simulink model "ProjektSim"  (R2018a)
settings: Solver=VariableStepAuto  StartTime=0.0  StopTime=50000  MaxStep=10  RelTol=1e-3
values from neighbouring files (symbols this model uses):
  Cp = 1000    [Projekt.m]
  Cvp = Cp * Rp * Vp    [Projekt.m]
  Cvw = Cp * Rp * Vw    [Projekt.m]
  Czas_skok = 5000    [Projekt.m]
  dFk = 0    [Projekt.m]
  dTg = -4    [Projekt.m]
  dTkz = 0    [Projekt.m]
  dTzew = -10    [Projekt.m]
  Fk0 = FkN    [Projekt.m]
  k1 = (Cp * Rp * FkN * (TkzN - TwewN) - kp * (TwewN - TpN)) / (TwewN - TzewN)    [Projekt.m]
  k2 = kp * (TwewN - TpN) / (TpN - TgN)    [Projekt.m]
  kp = Pr * Cp * Rp * FkN * (TkzN - TwewN) / (TwewN - TpN)    [Projekt.m]
  Rp = 1.2    [Projekt.m]
  Tg0 = TgN    (= -5)    [Projekt.m]
  Tkz0 = TkzN    (= 35)    [Projekt.m]
  Tp0 = (kp * Twew0 + k2 * Tg0) / (k2 + kp)    [Projekt.m]
  Twew0 = (Cp * Rp * Fk0 * Tkz0 + k1 * Tzew0 + k2 * kp * Tg0 / (k2 + kp)) / (Cp * Rp * Fk0 + k1 + kp - kp * kp / (k2 + kp))    [Projekt.m]
  Tzew0 = TzewN    (= -20)    [Projekt.m]
settings Model: Creator=aplov  LastModifiedBy=aplov

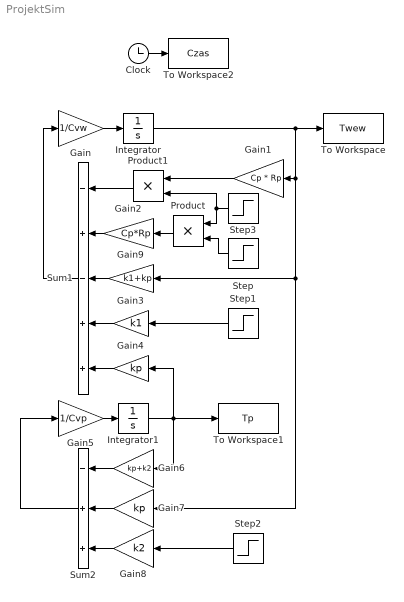
== system ProjektSim ==
  Clock : Clock
  Gain : Gain  Gain=1/Cvw
  Gain1 : Gain  Gain=Cp * Rp
  Gain2 : Gain  Gain=Cp*Rp
  Gain3 : Gain  Gain=k1
  Gain4 : Gain  Gain=kp
  Gain5 : Gain  Gain=1/Cvp
  Gain6 : Gain  Gain=kp+k2
  Gain7 : Gain  Gain=kp
  Gain8 : Gain  Gain=k2
  Gain9 : Gain  Gain=k1+kp
  Integrator : Integrator  InitialCondition=Twew0
  Integrator1 : Integrator  InitialCondition=Tp0
  Product : Product
  Product1 : Product
  Step : Step  Time=Czas_skok  Before=Tkz0  After=Tkz0 + dTkz  SampleTime=0
  Step1 : Step  Time=Czas_skok  Before=Tzew0  After=Tzew0 + dTzew  SampleTime=0
  Step2 : Step  Time=Czas_skok  Before=Tg0  After=Tg0 + dTg  SampleTime=0
  Step3 : Step  Time=Czas_skok  Before=Fk0  After=Fk0 + dFk  SampleTime=0
  Sum1 : Sum  Inputs=-+-++
  Sum2 : Sum  Inputs=-++
  To Workspace : ToWorkspace  VariableName=Twew  SampleTime=-1
  To Workspace1 : ToWorkspace  VariableName=Tp  SampleTime=-1
  To Workspace2 : ToWorkspace  VariableName=Czas  SampleTime=-1
  wires:
  Gain/1 -> Integrator/1
  Sum1/1 -> Gain/1
  Gain2/1 -> Sum1/2
  Gain3/1 -> Sum1/4
  Step1/1 -> Gain3/1
  Gain4/1 -> Sum1/5
  Integrator1/1 -> Gain6/1, To Workspace1/1, Gain4/1
  Gain5/1 -> Integrator1/1
  Sum2/1 -> Gain5/1
  Gain6/1 -> Sum2/1
  Gain7/1 -> Sum2/2
  Integrator/1 -> To Workspace/1, Gain7/1, Gain9/1, Gain1/1
  Gain8/1 -> Sum2/3
  Step2/1 -> Gain8/1
  Clock/1 -> To Workspace2/1
  Product/1 -> Gain2/1
  Step3/1 -> Product1/2, Product/1
  Step/1 -> Product/2
  Gain1/1 -> Product1/1
  Product1/1 -> Sum1/1
  Gain9/1 -> Sum1/3
